simulink model "Power_system_Noisy"  (R2017a)
settings: Solver=ode45  StartTime=0.0  StopTime=tsim  MaxStep=1e-4  RelTol=1e-3
values from neighbouring files (symbols this model uses):
  A2 = [0 1;0 0]    [Power_system_RZA_m.m]
  alpha = [alpha1;alpha0]    [Power_system_RZA_m.m]
  alpha0 = 1    [Power_system_RZA_m.m]
  B2 = [0;1]    [Power_system_RZA_m.m]
  C2 = [1 0]    [Power_system_RZA_m.m]
  Delta_f0 = 0    [Power_system_RZA_m.m]
  Delta_P0 = 0    [Power_system_RZA_m.m]
  Delta_X0 = 0.011    [Power_system_RZA_m.m]
  denC = conv([1 0],[tauC 1])    [Power_system_RZA_m.m]
  gn = -2*Klm/Tlm/Tg    (= -1.66666666667)    [Power_system_RZA_m.m]
  Gn = 3/Thn/Klm*(-1-Tlm/Thn)    (= -1.875)    [Power_system_RZA_m.m]
  Klm = 1    [Power_system_RZA_m.m]
  ks = -10    [Power_system_RZA_m.m]
  max_noise = 0.004    [Power_system_RZA_m.m]
  numC = [1.8124 -18.8558 0.1523]    [Power_system_RZA_m.m]
  ooverline_sat = overline_sat -1/ks    (= 20000.1)    [Power_system_RZA_m.m]
  overline_phin = [phin2; phin1]    [Power_system_RZA_m.m]
  overline_sat = 20000    [Power_system_RZA_m.m]
  psin = Klm/Tlm/Thn + Klm/Tlm/Tg    (= 0.875)    [Power_system_RZA_m.m]
  R = 0.05    [Power_system_RZA_m.m]
  Sn = 1/Thn    (= 0.25)    [Power_system_RZA_m.m]
  tau = 0.001    [Power_system_RZA_m.m]
  Tg = 0.2    [Power_system_RZA_m.m]
  Th2 = 6    [Power_system_RZA_m.m]
  Tlm = 6    [Power_system_RZA_m.m]
  ttrig = 60    [Power_system_RZA_m.m]
  underline_Delta = [tau 0;0 tau^2]    [Power_system_RZA_m.m]
  uunderline_sat = underline_sat + 1/ks    (= -20000.1)    [Power_system_RZA_m.m]
  zna0 = -0.001    [Power_system_RZA_m.m]
libraries: dspsrcs4 x1
settings Model: Creator=Gyunghoon  LastModifiedBy=Gyunghoon
settings DataIOCC: LimitDataPoints=on  SaveFormat=Array
settings OptimizationCC: BlockReduction=off  BooleanDataType=off  LifeSpan=inf
settings DebuggingCC: SaveWithParameterizedLinksMsg=none  UnderspecifiedInitializationDetection=Classic  MergeDetectMultiDrivingBlocksExec=none  SignalResolutionControl=TryResolveAllWithWarning  SFUnexpectedBacktrackingDiag=warning  SFNoUnconditionalDefaultTransitionDiag=warning  SFExecutionAtInitializationDiag=none
settings HardwareCC: ProdBitPerPointer=32  ProdBitPerSizeT=32  ProdBitPerPtrDiffT=32  ProdLargestAtomicFloat=None  ProdIntDivRoundTo=Undefined  ProdEndianess=Unspecified  ProdWordSize=32  ProdHWDeviceType=32-bit Generic  TargetUnknown=on
settings ModelReferenceCC: PropagateSignalLabelsOutOfModel=off
settings GRTTargetCC: TargetLangStandard=C89/C90 (ANSI)  GeneratePreprocessorConditionals=Disable all
settings ConfigComp: CovMetricSettings=dw  CovHtmlReporting=on  CovSaveCumulativeToWorkspaceVar=on  CovSaveSingleToWorkspaceVar=on  CovExternalEMLEnable=off  CovSFcnEnable=off

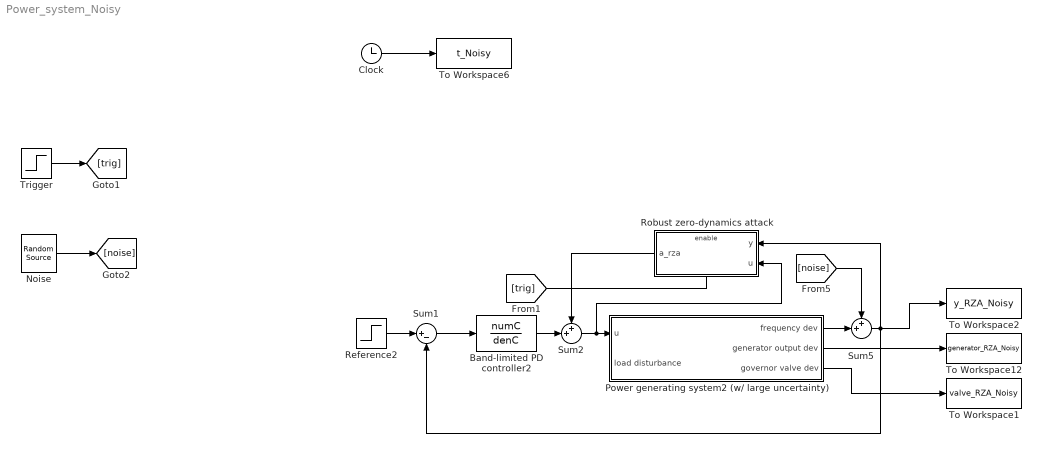
== system Power_system_Noisy ==
  Band-limited PD controller2 : TransferFcn  Numerator=numC  Denominator=denC
  Clock : Clock
  Noise : dspsrcs4/Random Source  SrcType=Uniform  NormMethod=Ziggurat  CltLength=12  MinVal=-max_noise  MaxVal=max_noise  MeanVal=0  VarVal=1  RepMode=Not repeatable  rawSeed=1  IsInherit=off  SampMode=Continuous  SampTime=1  SampFrame=1  DataType=Double  OutComplex=Real  OutputFrames=off
  Power generating system2 (w/ large uncertainty) : Subsystem
  Reference2 : Step  Time=0  After=0  SampleTime=0
  Robust zero-dynamics attack : Subsystem  TreatAsAtomicUnit=on
  Sum1 : Sum  Inputs=|+-
  Sum2 : Sum  Inputs=++|
  Sum5 : Sum  Inputs=++|
  To Workspace1 : ToWorkspace  VariableName=valve_RZA_Noisy  SampleTime=-1
  To Workspace12 : ToWorkspace  VariableName=generator_RZA_Noisy  SampleTime=-1
  To Workspace2 : ToWorkspace  VariableName=y_RZA_Noisy  SampleTime=-1
  To Workspace6 : ToWorkspace  VariableName=t_Noisy  SampleTime=-1
  Trigger : Step  Time=ttrig  SampleTime=0
  wires:
  Clock/1 -> To Workspace6/1
  Trigger/1 -> [trig]
  Sum1/1 -> Band-limited PD controller2/1
  Reference2/1 -> Sum1/1
  Band-limited PD controller2/1 -> Sum2/2
  Power generating system2 (w/ large uncertainty)/3(governor valve dev) -> To Workspace1/1
  Sum2/1 -> Robust zero-dynamics attack/2(u), Power generating system2 (w/ large uncertainty)/1(u)
  Robust zero-dynamics attack/1(a_rza) -> Sum2/1
  [trig] -> Robust zero-dynamics attack/Enable
  Power generating system2 (w/ large uncertainty)/2(generator output dev) -> To Workspace12/1
  Sum5/1 -> To Workspace2/1, Robust zero-dynamics attack/1(y), Sum1/2
  Noise/1 -> [noise]
  Power generating system2 (w/ large uncertainty)/1(frequency dev) -> Sum5/2
  [noise] -> Sum5/1

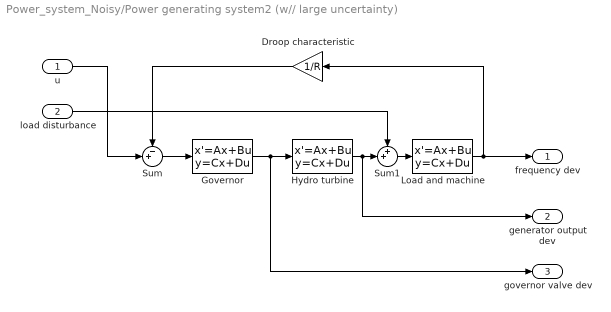
== system Power_system_Noisy/Power generating system2 (w// large uncertainty) ==
  u : Inport
  load disturbance : Inport  Port=2
  Droop characteristic : Gain  Gain=1/R
  Governor : StateSpace  A=-1/Tg  B=1/Tg  D=0  X0=Delta_X0
  Hydro turbine : StateSpace  A=-2/Th2  B=6/Th2  D=-2  X0=Delta_P0+2*Delta_X0
  Load and machine : StateSpace  A=-1/Tlm  B=Klm/Tlm  D=0  X0=Delta_f0
  Sum : Sum  Inputs=-+|
  Sum1 : Sum  Inputs=++|
  frequency dev : Outport
  generator output dev : Outport  Port=2
  governor valve dev : Outport  Port=3
  wires:
  u/1 -> Sum/2
  Droop characteristic/1 -> Sum/1
  Load and machine/1 -> Droop characteristic/1, frequency dev/1
  Hydro turbine/1 -> generator output dev/1, Sum1/2
  Sum/1 -> Governor/1
  Governor/1 -> Hydro turbine/1, governor valve dev/1
  Sum1/1 -> Load and machine/1
  load disturbance/1 -> Sum1/1

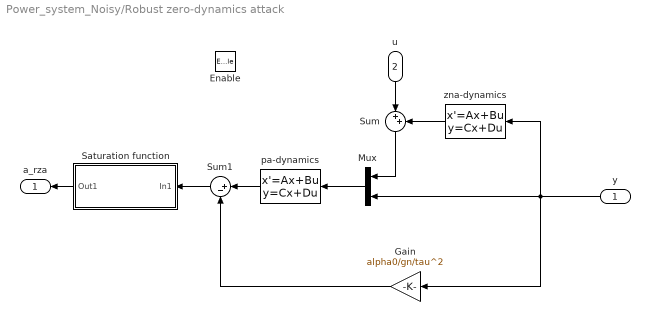
== system Power_system_Noisy/Robust zero-dynamics attack ==
  y : Inport
  u : Inport  Port=2
  Enable : EnablePort  PropagateVarSize=During execution
  Gain : Gain  Gain=alpha0/gn/tau^2
  Mux : Mux  Inputs=2
  Saturation function : Subsystem
  Sum : Sum  Inputs=|++
  Sum1 : Sum  Inputs=|+-
  pa-dynamics : StateSpace  A=A2-inv(underline_Delta)*alpha*C2  B=[alpha0/tau^2*B2 alpha0/tau^2/gn*(overline_phin+inv(underline_Delta)*alpha)]  C=C2  D=[0 0]  X0=[0 0]
  zna-dynamics : StateSpace  A=Sn  B=Gn  C=psin/gn  D=0  X0=zna0
  a_rza : Outport  OutputWhenDisabled=reset  InitialOutput=0
  wires:
  y/1 -> zna-dynamics/1, Gain/1, Mux/2
  Saturation function/1(Out1) -> a_rza/1
  Mux/1 -> pa-dynamics/1
  u/1 -> Sum/1
  zna-dynamics/1 -> Sum/2
  Sum/1 -> Mux/1
  pa-dynamics/1 -> Sum1/1
  Sum1/1 -> Saturation function/1(In1)
  Gain/1 -> Sum1/2

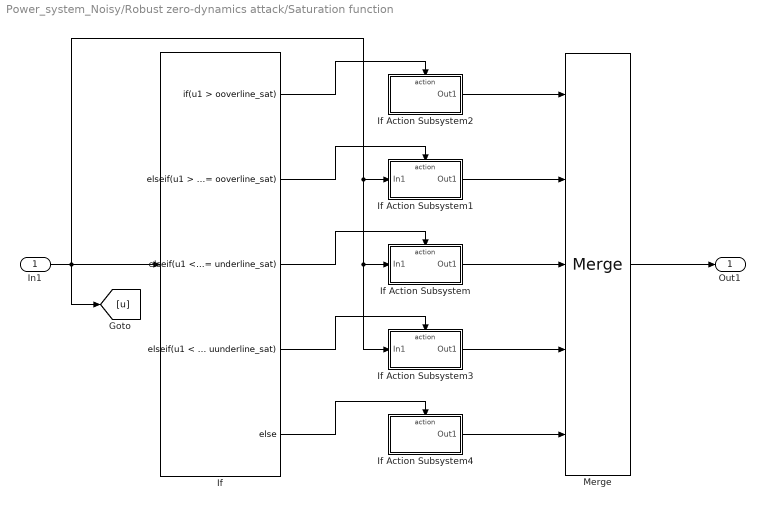
== system Power_system_Noisy/Robust zero-dynamics attack/Saturation function ==
  In1 : Inport
  If : If  IfExpression=u1 > ooverline_sat  ElseIfExpressions=u1 > overline_sat & u1 <= ooverline_sat, u1 <= overline_sat & u1>= underline_sat, u1 < underline_sat & u1 >= uunderline_sat
  If Action Subsystem : Subsystem  TreatAsAtomicUnit=on
  If Action Subsystem1 : Subsystem  TreatAsAtomicUnit=on
  If Action Subsystem2 : Subsystem  TreatAsAtomicUnit=on
  If Action Subsystem3 : Subsystem  TreatAsAtomicUnit=on
  If Action Subsystem4 : Subsystem  TreatAsAtomicUnit=on
  Merge : Merge  Inputs=5
  Out1 : Outport
  wires:
  In1/1 -> If Action Subsystem3/1(In1), If Action Subsystem/1(In1), If Action Subsystem1/1(In1), [u], If/1
  Merge/1 -> Out1/1
  If/3 -> If Action Subsystem/Action
  If Action Subsystem/1(Out1) -> Merge/3
  If/2 -> If Action Subsystem1/Action
  If Action Subsystem2/1(Out1) -> Merge/1
  If/1 -> If Action Subsystem2/Action
  If Action Subsystem3/1(Out1) -> Merge/4
  If/4 -> If Action Subsystem3/Action
  If Action Subsystem4/1(Out1) -> Merge/5
  If/5 -> If Action Subsystem4/Action
  If Action Subsystem1/1(Out1) -> Merge/2

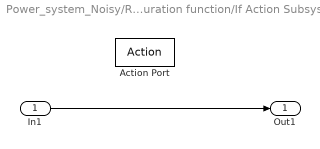
== system Power_system_Noisy/Robust zero-dynamics attack/Saturation function/If Action Subsystem ==
  In1 : Inport
  Action Port : ActionPort  ActionType=elseif
  Out1 : Outport
  wires:
  In1/1 -> Out1/1

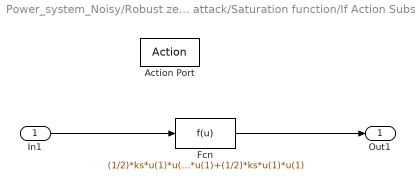
== system Power_system_Noisy/Robust zero-dynamics attack/Saturation function/If Action Subsystem1 ==
  In1 : Inport
  Action Port : ActionPort  ActionType=elseif
  Fcn : Fcn  Expr=(1/2)*ks*u(1)*u(1)+(-ks*overline_sat+1)*u(1)+(1/2)*ks*u(1)*u(1)
  Out1 : Outport
  wires:
  Fcn/1 -> Out1/1
  In1/1 -> Fcn/1

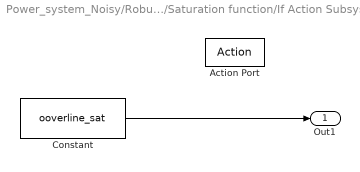
== system Power_system_Noisy/Robust zero-dynamics attack/Saturation function/If Action Subsystem2 ==
  Action Port : ActionPort  ActionType=then
  Constant : Constant  Value=ooverline_sat
  Out1 : Outport
  wires:
  Constant/1 -> Out1/1

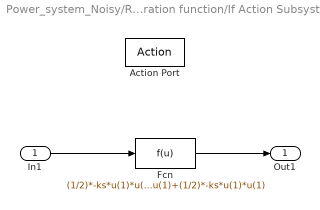
== system Power_system_Noisy/Robust zero-dynamics attack/Saturation function/If Action Subsystem3 ==
  In1 : Inport
  Action Port : ActionPort  ActionType=elseif
  Fcn : Fcn  Expr=(1/2)*-ks*u(1)*u(1)+(ks*overline_sat+1)*u(1)+(1/2)*-ks*u(1)*u(1)
  Out1 : Outport
  wires:
  Fcn/1 -> Out1/1
  In1/1 -> Fcn/1

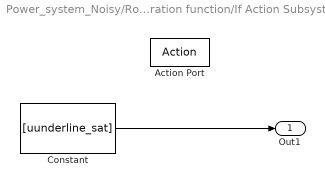
== system Power_system_Noisy/Robust zero-dynamics attack/Saturation function/If Action Subsystem4 ==
  Action Port : ActionPort  ActionType=else
  Constant : Constant  Value=[uunderline_sat]
  Out1 : Outport
  wires:
  Constant/1 -> Out1/1
